simulink model "Roboter_RRP_Sim"  (R2020b)
settings: Solver=ode15s  StartTime=0.0  StopTime=5  RelTol=1e-6  AbsTol=1e-5  EnableMultiTasking=on
InitFcn:
  | set_parameter
StartFcn:
  | set_parameter
undefined symbols (not defined in the file or in its folder): parReg, parSys, X, Y, Z
libraries: sm_lib x14, nesl_utility x4, fl_lib x1
settings Model: Creator=andreas  LastModifiedBy=ukn
settings SolverCC: AutoScaleAbsTol=off  MaxOrder=3
settings DataIOCC: LimitDataPoints=on  SaveFormat=Array  SignalLoggingSaveFormat=ModelDataLogs  ReturnWorkspaceOutputs=off
settings OptimizationCC: ExpressionDepthLimit=2147483647  InitFltsAndDblsToZero=on  LifeSpan=inf
settings DebuggingCC: SaveWithParameterizedLinksMsg=none  UnderspecifiedInitializationDetection=Classic  MergeDetectMultiDrivingBlocksExec=none  SignalResolutionControl=TryResolveAllWithWarning  SolverPrmCheckMsg=warning  MultiTaskDSMMsg=warning  MultiTaskCondExecSysMsg=none  FcnCallInpInsideContextMsg=warning  StateNameClashWarn=warning  SFUnexpectedBacktrackingDiag=warning  SFNoUnconditionalDefaultTransitionDiag=warning  SFExecutionAtInitializationDiag=none  ArithmeticOperatorsInVariantConditions=warning
settings HardwareCC: ProdBitPerPointer=32  ProdBitPerSizeT=32  ProdBitPerPtrDiffT=32  ProdLargestAtomicFloat=None  ProdIntDivRoundTo=Undefined  ProdEndianess=Unspecified  ProdWordSize=32  ProdHWDeviceType=32-bit Generic
settings ModelReferenceCC: PropagateSignalLabelsOutOfModel=off
settings SFSimCC: SimUseLocalCustomCode=off  CustomCodeUndefinedFunction=UseInterfaceOnly
settings RTWCC: RTWUseLocalCustomCode=off
settings CodeAppCC: StateflowObjectComments=on
settings GRTTargetCC: TargetFcnLib=ansi_tfl_tmw.mat  TargetLangStandard=C89/C90 (ANSI)  CombineOutputUpdateFcns=off  GRTInterface=on
settings ConfigComp: CovMetricSettings=dw  CovSaveCumulativeToWorkspaceVar=on  CovSaveSingleToWorkspaceVar=on  CovExternalEMLEnable=off

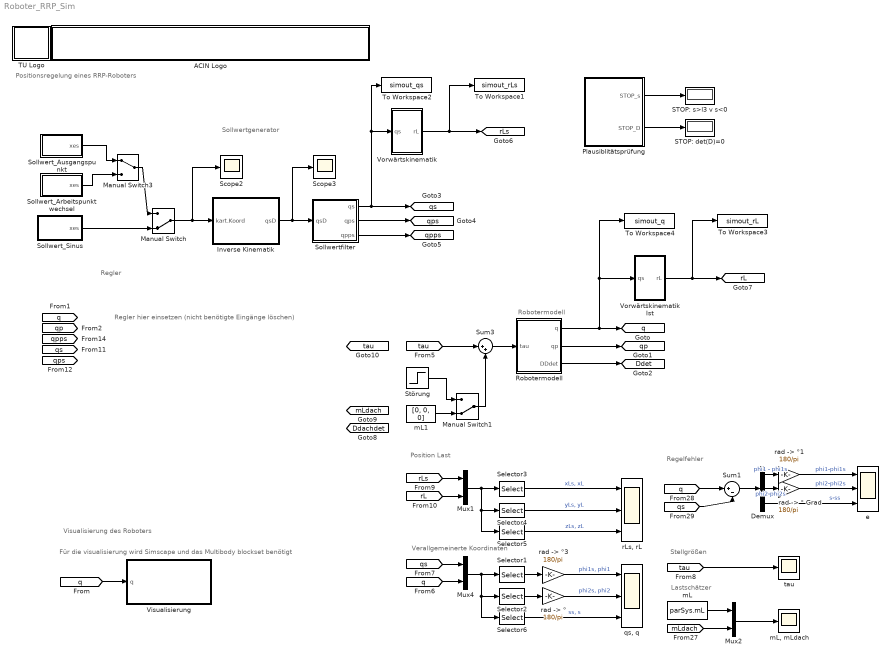
== system Roboter_RRP_Sim ==
  note: Positionsregelung eines RRP-Roboters
  note: Robotermodell
  note: Regler
  note: Sollwertgenerator
  note: Position Last
  note: Verallgemeinerte Koordinaten
  note: Regelfehler
  note: Stellgrößen
  note: Lastschätzer
  note: Regler
      | hier
      | einsetzen
      | (nicht benötigte Eingänge löschen)
  note: Für die visualisierung wird Simscape und das Multibody blockset benötigt
  note: Visualisierung des Roboters
  ACIN Logo : Subsystem
      mask init:
      | s = get_param(gcb,'UserData');
      mask Display:
      | image(s.logo,[0 0 439 45]);
      | %axis image
  Demux : Demux  Outputs=3
  Inverse Kinematik : Subsystem
  Manual Switch : ManualSwitch  CurrentSetting=0
  Manual Switch1 : ManualSwitch  CurrentSetting=0
  Manual Switch3 : ManualSwitch
  Mux1 : Mux  Inputs=2
  Mux2 : Mux  Inputs=2
  Mux4 : Mux  Inputs=2
  Plausiblitätsprüfung : Subsystem
  Robotermodell : Subsystem
  STOP: det(D)=0 : Display
  STOP: s>l3 v s<0 : Display
  Scope2 : Scope
  Scope3 : Scope
  Selector1 : Selector  InputPortWidth=6  IndexOptions=Index vector (dialog)  Indices=[1 4]  OutputSizes=1
  Selector2 : Selector  InputPortWidth=6  IndexOptions=Index vector (dialog)  Indices=[2 5]  OutputSizes=1
  Selector3 : Selector  InputPortWidth=6  IndexOptions=Index vector (dialog)  Indices=[1 4]  OutputSizes=1
  Selector4 : Selector  InputPortWidth=6  IndexOptions=Index vector (dialog)  Indices=[2 5]  OutputSizes=1
  Selector5 : Selector  InputPortWidth=6  IndexOptions=Index vector (dialog)  Indices=[3 6]  OutputSizes=1
  Selector6 : Selector  InputPortWidth=6  IndexOptions=Index vector (dialog)  Indices=[3 6]  OutputSizes=1
  Sollwert_Arbeitspunktwechsel : Subsystem
  Sollwert_Ausgangspunkt : Subsystem
  Sollwert_Sinus : Subsystem
  Sollwertfilter : Subsystem
  Störung : Step  After=[250, 250, 200]  SampleTime=0
  Sum1 : Sum  Inputs=|+-
  Sum3 : Sum  Inputs=|++
  TU Logo : Subsystem
      mask init:
      | s = get_param(gcb,'UserData');
      mask Display: image(s.logo,[0 0 45 45]);
  To Workspace1 : ToWorkspace  VariableName=simout_rLs  SaveFormat=Structure With Time  SampleTime=-1
  To Workspace2 : ToWorkspace  VariableName=simout_qs  SaveFormat=Structure With Time  SampleTime=-1
  To Workspace3 : ToWorkspace  VariableName=simout_rL  SaveFormat=Structure With Time  SampleTime=-1
  To Workspace4 : ToWorkspace  VariableName=simout_q  SaveFormat=Structure With Time  SampleTime=-1
  Visualisierung : Subsystem
  Vorwärtskinematik : Subsystem
  Vorwärtskinematik Ist : Subsystem
  e : Scope  NumInputPorts=3
  mL : Constant  Value=parSys.mL
  "mL, mLdach" : Scope
  mL1 : Constant  Value=[0, 0, 0]
  "qs, q" : Scope  NumInputPorts=3
  "rLs, rL" : Scope  NumInputPorts=3
  "rad -> °" : Gain  Gain=180/pi
  "rad -> ° Grad" : Gain  Gain=180/pi
  "rad -> °1" : Gain  Gain=180/pi
  "rad -> °3" : Gain  Gain=180/pi
  tau : Scope
  tag scope: Ddachdet=global, Ddet=global, mLdach=global, q=global, qp=global, qpps=global, qps=global, qs=global, rL=global, rLs=global, tau=global
  wires:
  Robotermodell/1(q) -> Vorwärtskinematik Ist/1(qs), To Workspace4/1, [q]
  Robotermodell/2(qp) -> [qp]
  Inverse Kinematik/1(qsD) -> Scope3/1, Sollwertfilter/1(qsD)
  [tau] -> tau/1
  Vorwärtskinematik Ist/1(rL) -> [rL], To Workspace3/1
  Manual Switch/1 -> Inverse Kinematik/1(kart.Koord), Scope2/1
  Sollwert_Sinus/1(xes) -> Manual Switch/2
  [qs] -> Mux4/1
  [q] -> Mux4/2
  Mux4/1 -> Selector1/1, Selector2/1, Selector6/1
  [rLs] -> Mux1/1
  [rL] -> Mux1/2
  Selector3/1 -> "rLs, rL"/1  "xLs, xL"
  Selector4/1 -> "rLs, rL"/2  "yLs, yL"
  Selector5/1 -> "rLs, rL"/3  "zLs, zL"
  Mux1/1 -> Selector5/1, Selector4/1, Selector3/1
  Manual Switch3/1 -> Manual Switch/1
  Sollwert_Arbeitspunktwechsel/1(xes) -> Manual Switch3/2
  Sollwert_Ausgangspunkt/1(xes) -> Manual Switch3/1
  Plausiblitätsprüfung/1(STOP_s) -> STOP: s>l3 v s<0/1
  Sollwertfilter/1(qs) -> [qs], Vorwärtskinematik/1(qs), To Workspace2/1
  Sollwertfilter/3(qpps) -> [qpps]
  Sollwertfilter/2(qps) -> [qps]
  [q] -> Sum1/1
  Demux/1 -> "rad -> °1"/1  "phi1 - phi1s"
  Demux/2 -> "rad -> ° Grad"/1  "phi2-phi2s"
  Demux/3 -> e/3  "s-ss"
  [qs] -> Sum1/2
  Sum1/1 -> Demux/1
  [tau] -> Sum3/1
  Sum3/1 -> Robotermodell/1(tau)
  Störung/1 -> Manual Switch1/1
  mL1/1 -> Manual Switch1/2
  Manual Switch1/1 -> Sum3/2
  Mux2/1 -> "mL, mLdach"/1
  mL/1 -> Mux2/1
  [mLdach] -> Mux2/2
  Selector1/1 -> "rad -> °3"/1
  Selector2/1 -> "rad -> °"/1
  Selector6/1 -> "qs, q"/3  "ss, s"
  "rad -> °"/1 -> "qs, q"/2  "phi2s, phi2"
  "rad -> °3"/1 -> "qs, q"/1  "phi1s, phi1"
  "rad -> °1"/1 -> e/1  "phi1-phi1s"
  "rad -> ° Grad"/1 -> e/2  "phi2-phi2s"
  Vorwärtskinematik/1(rL) -> [rLs], To Workspace1/1
  Plausiblitätsprüfung/2(STOP_D) -> STOP: det(D)=0/1
  Robotermodell/3(DDdet) -> [Ddet]
  [q] -> Visualisierung/1(q)

== system Roboter_RRP_Sim/ACIN Logo ==

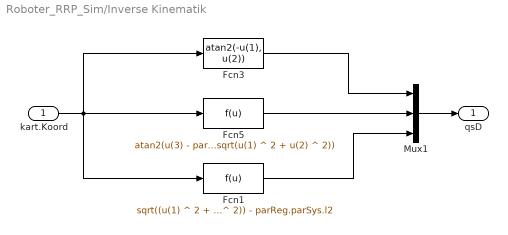
== system Roboter_RRP_Sim/Inverse Kinematik ==
  kart.Koord : Inport
  Fcn1 : Fcn  Expr=sqrt((u(1) ^ 2 + u(2) ^ 2 + u(3) ^ 2 - 2 * u(3) * parReg.parSys.l1 + parReg.parSys.l1 ^ 2)) - parReg.parSys.l2
  Fcn3 : Fcn  Expr=atan2(-u(1), u(2))
  Fcn5 : Fcn  Expr=atan2(u(3) - parReg.parSys.l1, sqrt(u(1) ^ 2 + u(2) ^ 2))
  Mux1 : Mux  Inputs=3
  qsD : Outport
  wires:
  kart.Koord/1 -> Fcn3/1, Fcn1/1, Fcn5/1
  Fcn3/1 -> Mux1/1
  Fcn5/1 -> Mux1/2
  Mux1/1 -> qsD/1
  Fcn1/1 -> Mux1/3

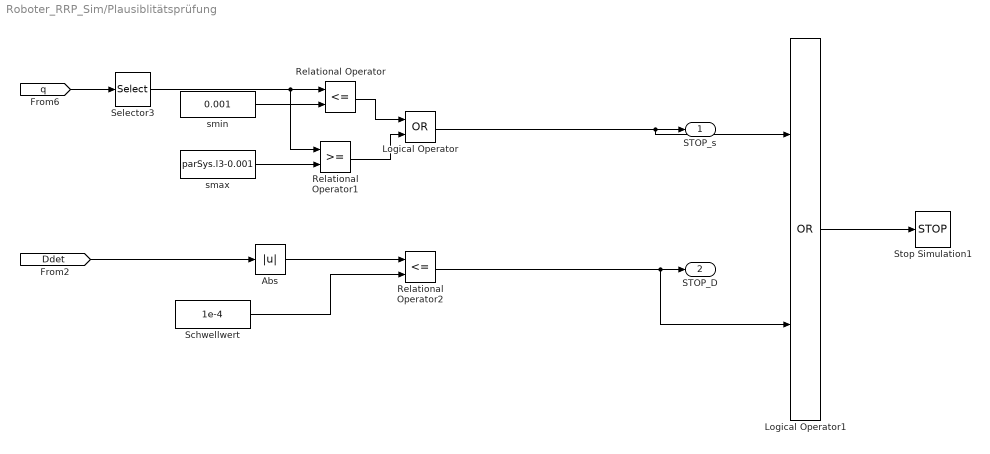
== system Roboter_RRP_Sim/Plausiblitätsprüfung ==
  Abs : Abs
  Logical Operator : Logic  Operator=OR  AllPortsSameDT=off  OutDataTypeStr=boolean
  Logical Operator1 : Logic  Operator=OR  AllPortsSameDT=off  OutDataTypeStr=boolean
  Relational Operator : RelationalOperator  Operator=<=  OutDataTypeStr=boolean  RndMeth=Nearest
  Relational Operator1 : RelationalOperator  OutDataTypeStr=boolean  RndMeth=Nearest
  Relational Operator2 : RelationalOperator  Operator=<=  OutDataTypeStr=boolean  RndMeth=Nearest
  Schwellwert : Constant  Value=1e-4
  Selector3 : Selector  InputPortWidth=3  IndexOptions=Index vector (dialog)  Indices=[3]  OutputSizes=1
  Stop Simulation1 : Stop
  smax : Constant  Value=parSys.l3-0.001
  smin : Constant  Value=0.001
  STOP_s : Outport
  STOP_D : Outport  Port=2
  wires:
  Relational Operator/1 -> Logical Operator/1
  Relational Operator1/1 -> Logical Operator/2
  [q] -> Selector3/1
  Selector3/1 -> Relational Operator/1, Relational Operator1/1
  smin/1 -> Relational Operator/2
  [Ddet] -> Abs/1
  Abs/1 -> Relational Operator2/1
  Schwellwert/1 -> Relational Operator2/2
  Logical Operator1/1 -> Stop Simulation1/1
  smax/1 -> Relational Operator1/2
  Relational Operator2/1 -> STOP_D/1, Logical Operator1/2
  Logical Operator/1 -> STOP_s/1, Logical Operator1/1

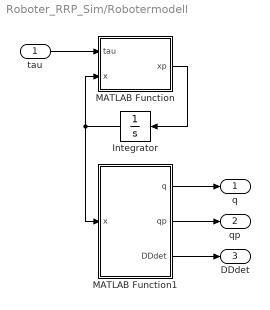
== system Roboter_RRP_Sim/Robotermodell ==
  tau : Inport
  Integrator : Integrator  InitialCondition=[parSys.phi10; parSys.phi20; parSys.s0; parSys.phi1p0; parSys.phi2p0; parSys.sp0]
  MATLAB Function : MATLAB Function  TreatAsAtomicUnit=on
  MATLAB Function1 : MATLAB Function  TreatAsAtomicUnit=on
  q : Outport
  qp : Outport  Port=2
  DDdet : Outport  Port=3
  wires:
  MATLAB Function1/2(qp) -> qp/1
  MATLAB Function/1(xp) -> Integrator/1
  MATLAB Function1/3(DDdet) -> DDdet/1
  Integrator/1 -> MATLAB Function1/1(x), MATLAB Function/2(x)
  tau/1 -> MATLAB Function/1(tau)
  MATLAB Function1/1(q) -> q/1

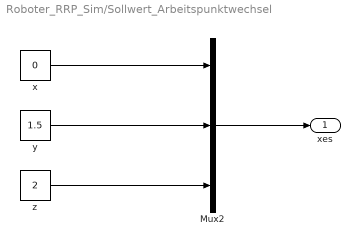
== system Roboter_RRP_Sim/Sollwert_Arbeitspunktwechsel ==
  Mux2 : Mux  Inputs=3
  x : Constant  Value=0
  y : Constant  Value=1.5
  z : Constant  Value=2
  xes : Outport
  wires:
  Mux2/1 -> xes/1
  x/1 -> Mux2/1
  y/1 -> Mux2/2
  z/1 -> Mux2/3

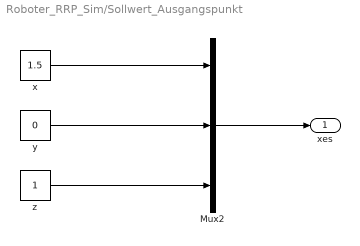
== system Roboter_RRP_Sim/Sollwert_Ausgangspunkt ==
  Mux2 : Mux  Inputs=3
  x : Constant  Value=1.5
  y : Constant  Value=0
  z : Constant
  xes : Outport
  wires:
  z/1 -> Mux2/3
  y/1 -> Mux2/2
  x/1 -> Mux2/1
  Mux2/1 -> xes/1

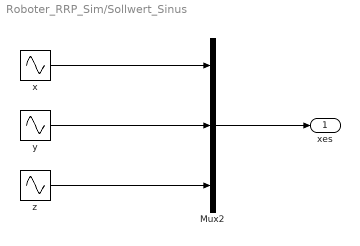
== system Roboter_RRP_Sim/Sollwert_Sinus ==
  Mux2 : Mux  Inputs=3
  x : Sin  Amplitude=1.5  Frequency=2*pi*parReg.traj_fKreis  Phase=pi/2  SampleTime=0
  y : Sin  Amplitude=1.5  Frequency=2*pi*parReg.traj_fKreis  SampleTime=0
  z : Sin  Amplitude=0.5  Bias=1.5  Frequency=2*pi*parReg.traj_fz  Phase=-pi/2  SampleTime=0
  xes : Outport
  wires:
  Mux2/1 -> xes/1
  x/1 -> Mux2/1
  y/1 -> Mux2/2
  z/1 -> Mux2/3

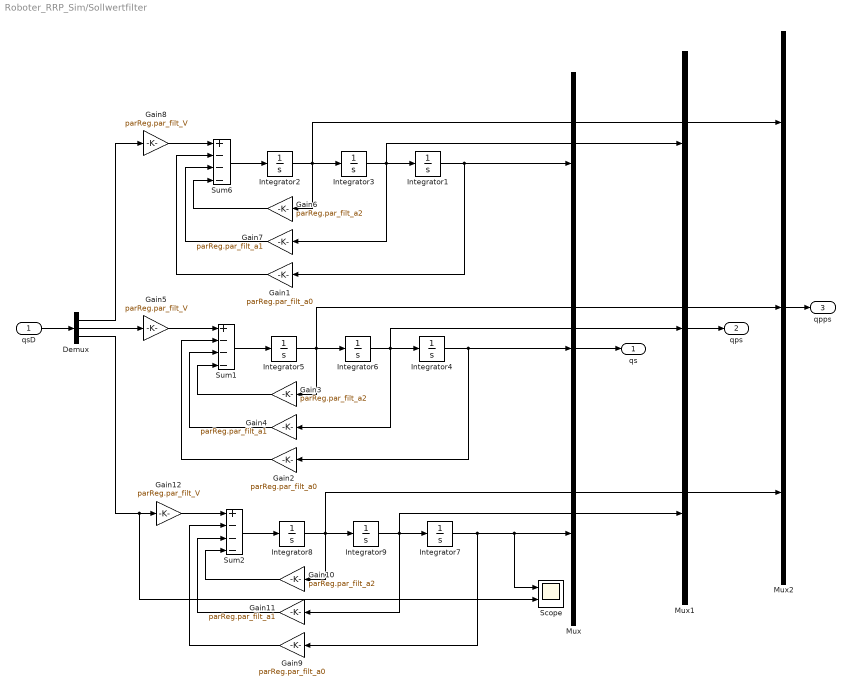
== system Roboter_RRP_Sim/Sollwertfilter ==
  qsD : Inport
  Demux : Demux  Outputs=3
  Gain1 : Gain  Gain=parReg.par_filt_a0  SaturateOnIntegerOverflow=on  OutDataTypeStr=Inherit: Same as input  ParamDataTypeStr=Inherit: Same as input
  Gain10 : Gain  Gain=parReg.par_filt_a2  SaturateOnIntegerOverflow=on  OutDataTypeStr=Inherit: Same as input  ParamDataTypeStr=Inherit: Same as input
  Gain11 : Gain  Gain=parReg.par_filt_a1  SaturateOnIntegerOverflow=on  OutDataTypeStr=Inherit: Same as input  ParamDataTypeStr=Inherit: Same as input
  Gain12 : Gain  Gain=parReg.par_filt_V  SaturateOnIntegerOverflow=on  OutDataTypeStr=Inherit: Same as input  ParamDataTypeStr=Inherit: Same as input
  Gain2 : Gain  Gain=parReg.par_filt_a0  SaturateOnIntegerOverflow=on  OutDataTypeStr=Inherit: Same as input  ParamDataTypeStr=Inherit: Same as input
  Gain3 : Gain  Gain=parReg.par_filt_a2  SaturateOnIntegerOverflow=on  OutDataTypeStr=Inherit: Same as input  ParamDataTypeStr=Inherit: Same as input
  Gain4 : Gain  Gain=parReg.par_filt_a1  SaturateOnIntegerOverflow=on  OutDataTypeStr=Inherit: Same as input  ParamDataTypeStr=Inherit: Same as input
  Gain5 : Gain  Gain=parReg.par_filt_V  SaturateOnIntegerOverflow=on  OutDataTypeStr=Inherit: Same as input  ParamDataTypeStr=Inherit: Same as input
  Gain6 : Gain  Gain=parReg.par_filt_a2  SaturateOnIntegerOverflow=on  OutDataTypeStr=Inherit: Same as input  ParamDataTypeStr=Inherit: Same as input
  Gain7 : Gain  Gain=parReg.par_filt_a1  SaturateOnIntegerOverflow=on  OutDataTypeStr=Inherit: Same as input  ParamDataTypeStr=Inherit: Same as input
  Gain8 : Gain  Gain=parReg.par_filt_V  SaturateOnIntegerOverflow=on  OutDataTypeStr=Inherit: Same as input  ParamDataTypeStr=Inherit: Same as input
  Gain9 : Gain  Gain=parReg.par_filt_a0  SaturateOnIntegerOverflow=on  OutDataTypeStr=Inherit: Same as input  ParamDataTypeStr=Inherit: Same as input
  Integrator1 : Integrator  InitialCondition=parReg.traj_phi10
  Integrator{2..3,5..6,8..9} (6 alike) : Integrator
  Integrator4 : Integrator  InitialCondition=parReg.traj_phi20
  Integrator7 : Integrator  InitialCondition=parReg.traj_s0
  Mux : Mux  Inputs=3
  Mux1 : Mux  Inputs=3
  Mux2 : Mux  Inputs=3
  Scope : Scope  NumInputPorts=2
  Sum1 : Sum  Inputs=+---  InputSameDT=on  SaturateOnIntegerOverflow=on  OutDataTypeStr=Inherit: Same as first input
  Sum2 : Sum  Inputs=+---  InputSameDT=on  SaturateOnIntegerOverflow=on  OutDataTypeStr=Inherit: Same as first input
  Sum6 : Sum  Inputs=+---  InputSameDT=on  SaturateOnIntegerOverflow=on  OutDataTypeStr=Inherit: Same as first input
  qs : Outport
  qps : Outport  Port=2
  qpps : Outport  Port=3
  wires:
  Mux/1 -> qs/1
  qsD/1 -> Demux/1
  Demux/1 -> Gain8/1
  Sum6/1 -> Integrator2/1
  Gain8/1 -> Sum6/1
  Integrator3/1 -> Integrator1/1, Gain7/1, Mux1/1
  Integrator2/1 -> Integrator3/1, Gain6/1, Mux2/1
  Integrator1/1 -> Gain1/1, Mux/1
  Gain6/1 -> Sum6/4
  Gain7/1 -> Sum6/3
  Gain1/1 -> Sum6/2
  Sum1/1 -> Integrator5/1
  Gain5/1 -> Sum1/1
  Integrator6/1 -> Gain4/1, Integrator4/1, Mux1/2
  Integrator5/1 -> Gain3/1, Integrator6/1, Mux2/2
  Integrator4/1 -> Gain2/1, Mux/2
  Gain3/1 -> Sum1/4
  Gain4/1 -> Sum1/3
  Gain2/1 -> Sum1/2
  Demux/2 -> Gain5/1
  Sum2/1 -> Integrator8/1
  Gain12/1 -> Sum2/1
  Integrator9/1 -> Integrator7/1, Gain11/1, Mux1/3
  Integrator8/1 -> Integrator9/1, Gain10/1, Mux2/3
  Integrator7/1 -> Gain9/1, Mux/3, Scope/1
  Gain10/1 -> Sum2/4
  Gain11/1 -> Sum2/3
  Gain9/1 -> Sum2/2
  Demux/3 -> Gain12/1, Scope/2
  Mux1/1 -> qps/1
  Mux2/1 -> qpps/1

== system Roboter_RRP_Sim/TU Logo ==

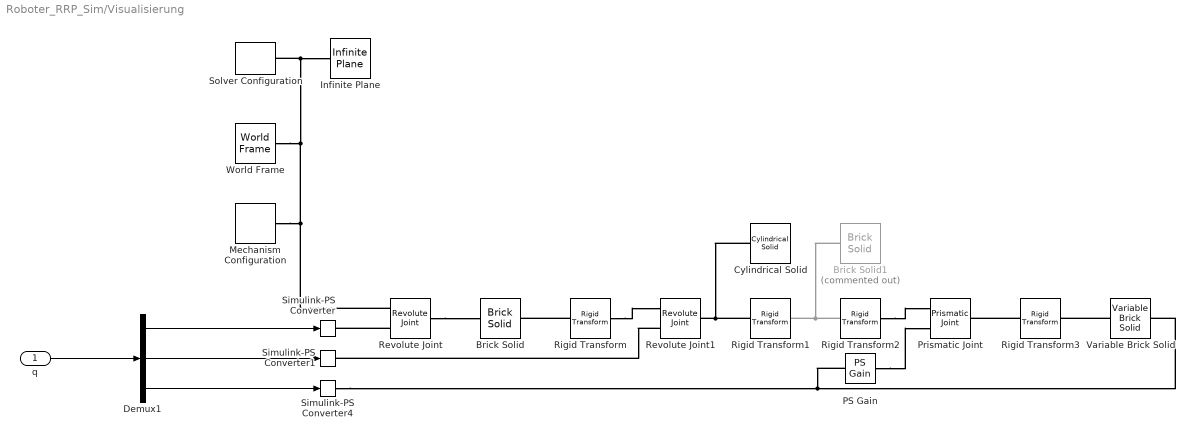
== system Roboter_RRP_Sim/Visualisierung ==
  q : Inport
  Brick Solid : sm_lib/Body Elements/Brick Solid  GraphicAmbientColor=[0.15 0.15 0.15 1.0]  BasedOnType=Density  BrickDimensions=[.1 .05 1]  BrickDimensionUnits=m  CenterOfMass=[0 0 0]  CenterOfMassUnits=m  GraphicDiffuseColor=[0.5 0.5 0.5]  Density=1000  DensityUnits=kg/m^3  DoExposeReferenceFrame=off  GraphicEmissiveColor=[0.0 0.0 0.0 1.0]  ExportEntireGeometry=off  SerializedFrames=<Frames><Frame><Id>Frame1</Id><Value><Name>F1</Name><Origin><Source>GeometricFeature</Source><FeatureName>-z surface</FeatureName></Origin><PrimaryAxis><DefinedDirection>+Z</DefinedDirection><Source>ReferenceFrame</Source><SourceDirection>+Z</SourceDirection><FeatureName></FeatureName></PrimaryAxis><SecondaryAxis><DefinedDirection>+X</DefinedDirection><Source>ReferenceFrame</Source><SourceDirection>+X</SourceDirection><FeatureName></FeatureName></SecondaryAxis></Value></Frame><Frame><Id>Frame2</Id><Value><Name>F2</Name><Origin><Source>GeometricFeature</Source><FeatureName>+z surface</FeatureName></Origin><PrimaryAxis><DefinedDirection>+Z</DefinedDirection><Source>ReferenceFrame</Source><SourceDirection>+Z</SourceDirection><FeatureName></FeatureName></PrimaryAxis><SecondaryAxis><DefinedDirection>+X</DefinedDirection><Source>ReferenceFrame</Source><SourceDirection>+X</SourceDirection><FeatureName></FeatureName></SecondaryAxis></Value></Frame></Frames>  MarkerShape=Sphere  MarkerSize=10  GraphicType=FromGeometry  InertiaType=CalculateFromGeometry  Mass=1  MassUnits=kg  MomentsOfInertia=[1 1 1]  MomentsOfInertiaUnits=kg*m^2  GraphicOpacity=1.0  ProductsOfInertia=[0 0 0]  ProductsOfInertiaUnits=kg*m^2  GraphicShininess=75  GraphicSpecularColor=[0.5 0.5 0.5 1.0]  GraphicVisPropType=SimpleVisualProperties
  Brick Solid1 : sm_lib/Body Elements/Brick Solid  Commented=on  GraphicAmbientColor=[0.15 0.15 0.15 1.0]  BasedOnType=Density  BrickDimensions=[.1 .5 .05]  BrickDimensionUnits=m  CenterOfMass=[0 0 0]  CenterOfMassUnits=m  GraphicDiffuseColor=[0.5 0.5 0.5]  Density=1000  DensityUnits=kg/m^3  DoExposeReferenceFrame=off  GraphicEmissiveColor=[0.0 0.0 0.0 1.0]  ExportEntireGeometry=off  SerializedFrames=<Frames><Frame><Id>Frame1</Id><Value><Name>F1</Name><Origin><Source>GeometricFeature</Source><FeatureName>-y surface</FeatureName></Origin><PrimaryAxis><DefinedDirection>+Z</DefinedDirection><Source>ReferenceFrame</Source><SourceDirection>+Z</SourceDirection><FeatureName></FeatureName></PrimaryAxis><SecondaryAxis><DefinedDirection>+X</DefinedDirection><Source>ReferenceFrame</Source><SourceDirection>+X</SourceDirection><FeatureName></FeatureName></SecondaryAxis></Value></Frame><Frame><Id>Frame2</Id><Value><Name>F2</Name><Origin><Source>GeometricFeature</Source><FeatureName>+y surface</FeatureName></Origin><PrimaryAxis><DefinedDirection>+Z</DefinedDirection><Source>ReferenceFrame</Source><SourceDirection>+Z</SourceDirection><FeatureName></FeatureName></PrimaryAxis><SecondaryAxis><DefinedDirection>+X</DefinedDirection><Source>ReferenceFrame</Source><SourceDirection>+X</SourceDirection><FeatureName></FeatureName></SecondaryAxis></Value></Frame></Frames>  MarkerShape=Sphere  MarkerSize=10  GraphicType=FromGeometry  InertiaType=CalculateFromGeometry  Mass=1  MassUnits=kg  MomentsOfInertia=[1 1 1]  MomentsOfInertiaUnits=kg*m^2  GraphicOpacity=1.0  ProductsOfInertia=[0 0 0]  ProductsOfInertiaUnits=kg*m^2  GraphicShininess=75  GraphicSpecularColor=[0.5 0.5 0.5 1.0]  GraphicVisPropType=SimpleVisualProperties
  Cylindrical Solid : sm_lib/Body Elements/Cylindrical Solid  GraphicAmbientColor=[0.15 0.15 0.15 1.0]  BasedOnType=Density  CenterOfMass=[0 0 0]  CenterOfMassUnits=m  GraphicDiffuseColor=[0.5 0.5 0.5]  CylinderLength=.1  CylinderLengthUnits=m  CylinderRadius=.05  CylinderRadiusUnits=m  Density=1000  DensityUnits=kg/m^3  DoExposeReferenceFrame=on  GraphicEmissiveColor=[0.0 0.0 0.0 1.0]  ExportEntireGeometry=off  SerializedFrames=<Frames/>  MarkerShape=Sphere  MarkerSize=10  GraphicType=FromGeometry  InertiaType=CalculateFromGeometry  Mass=1  MassUnits=kg  MomentsOfInertia=[1 1 1]  MomentsOfInertiaUnits=kg*m^2  GraphicOpacity=1.0  ProductsOfInertia=[0 0 0]  ProductsOfInertiaUnits=kg*m^2  GraphicShininess=75  GraphicSpecularColor=[0.5 0.5 0.5 1.0]  GraphicVisPropType=SimpleVisualProperties
  Demux1 : Demux  Outputs=3
  Infinite Plane : sm_lib/Curves and Surfaces/Infinite Plane  GraphicType=Rectangle  GraphicPlaneWidth=1  GraphicPlaneWidthUnits=m  GraphicPlaneHeight=1  GraphicPlaneHeightUnits=m  GraphicVisPropType=SimpleVisualProperties  GraphicDiffuseColor=[0.5 0.5 0.5]  GraphicOpacity=0.25  GraphicSpecularColor=[0.5 0.5 0.5 1.0]  GraphicAmbientColor=[0.15 0.15 0.15 1.0]  GraphicEmissiveColor=[0.0 0.0 0.0 1.0]  GraphicShininess=75
  Mechanism Configuration : sm_lib/Utilities/Mechanism Configuration  UniformGravity=Constant  GravityVector=[0 0 0]  GravityVectorUnits=m/s^2  GravityUnits=m/s^2  LinearizationDelta=0.001  JointModeTransitionNonlinearIterations=2
  PS Gain : fl_lib/Physical Signals/Functions/PS Gain  gain=.5
  Prismatic Joint : sm_lib/Joints/Prismatic Joint  JointMode=Normal  SenseConstraintForce=off  SenseConstraintForceX=off  SenseConstraintForceY=off  SenseConstraintForceZ=off  SenseConstraintTorque=off  SenseConstraintTorqueX=off  SenseConstraintTorqueY=off  SenseConstraintTorqueZ=off  SenseTotalForce=off  SenseTotalForceX=off  SenseTotalForceY=off  SenseTotalForceZ=off  SenseTotalTorque=off  SenseTotalTorqueX=off  SenseTotalTorqueY=off  SenseTotalTorqueZ=off  CompositeWrenchDir=FollowerOnBase  CompositeWrenchFrame=BaseFrame  EquilibriumPosition=0  EquilibriumPositionUnits=m  SpringStiffness=0  SpringStiffnessUnits=N/m  DampingCoefficient=0  DampingCoefficientUnits=N/(m/s)  TorqueActuationMode=ComputedTorque  MotionActuationMode=InputMotion  SensePosition=off  SenseVelocity=off  SenseAcceleration=off  SenseTorqueForce=off  SenseLowerLimitTorqueForce=off  SenseUpperLimitTorqueForce=off  LowerLimitSpecify=off  LowerLimitBound=-1  LowerLimitBoundUnits=m  LowerLimitStiffness=1e6  LowerLimitStiffnessUnits=N/m  LowerLimitDamping=1e3  LowerLimitDampingUnits=N/(m/s)  LowerLimitTransitionRegionWidth=1e-4  LowerLimitTransitionRegionWidthUnits=m  UpperLimitSpecify=off  UpperLimitBound=1  UpperLimitBoundUnits=m  UpperLimitStiffness=1e6  UpperLimitStiffnessUnits=N/m  UpperLimitDamping=1e3  UpperLimitDampingUnits=N/(m/s)  UpperLimitTransitionRegionWidth=1e-4  UpperLimitTransitionRegionWidthUnits=m  PositionTargetSpecify=off  PositionTargetPriority=High  PositionTargetValue=0  PositionTargetValueUnits=m  VelocityTargetSpecify=off  VelocityTargetPriority=High  VelocityTargetValue=0  VelocityTargetValueUnits=m/s
  Revolute Joint : sm_lib/Joints/Revolute Joint  JointMode=Normal  SenseConstraintForce=off  SenseConstraintForceX=off  SenseConstraintForceY=off  SenseConstraintForceZ=off  SenseConstraintTorque=off  SenseConstraintTorqueX=off  SenseConstraintTorqueY=off  SenseConstraintTorqueZ=off  SenseTotalForce=off  SenseTotalForceX=off  SenseTotalForceY=off  SenseTotalForceZ=off  SenseTotalTorque=off  SenseTotalTorqueX=off  SenseTotalTorqueY=off  SenseTotalTorqueZ=off  CompositeWrenchDir=FollowerOnBase  CompositeWrenchFrame=BaseFrame  EquilibriumPosition=0  EquilibriumPositionUnits=deg  SpringStiffness=0  SpringStiffnessUnits=N*m/deg  DampingCoefficient=0  DampingCoefficientUnits=N*m/(deg/s)  TorqueActuationMode=ComputedTorque  MotionActuationMode=InputMotion  SensePosition=off  SenseVelocity=off  SenseAcceleration=off  SenseTorqueForce=off  SenseLowerLimitTorqueForce=off  SenseUpperLimitTorqueForce=off  LowerLimitSpecify=off  LowerLimitBound=-90  LowerLimitBoundUnits=deg  LowerLimitStiffness=1e4  LowerLimitStiffnessUnits=N*m/deg  LowerLimitDamping=10  LowerLimitDampingUnits=N*m/(deg/s)  LowerLimitTransitionRegionWidth=0.1  LowerLimitTransitionRegionWidthUnits=deg  UpperLimitSpecify=off  UpperLimitBound=90  UpperLimitBoundUnits=deg  UpperLimitStiffness=1e4  UpperLimitStiffnessUnits=N*m/deg  UpperLimitDamping=10  UpperLimitDampingUnits=N*m/(deg/s)  UpperLimitTransitionRegionWidth=0.1  UpperLimitTransitionRegionWidthUnits=deg  PositionTargetSpecify=off  PositionTargetPriority=High  PositionTargetValue=0  PositionTargetValueUnits=deg  VelocityTargetSpecify=off  VelocityTargetPriority=High  VelocityTargetValue=0  VelocityTargetValueUnits=deg/s
  Revolute Joint1 : sm_lib/Joints/Revolute Joint  JointMode=Normal  SenseConstraintForce=off  SenseConstraintForceX=off  SenseConstraintForceY=off  SenseConstraintForceZ=off  SenseConstraintTorque=off  SenseConstraintTorqueX=off  SenseConstraintTorqueY=off  SenseConstraintTorqueZ=off  SenseTotalForce=off  SenseTotalForceX=off  SenseTotalForceY=off  SenseTotalForceZ=off  SenseTotalTorque=off  SenseTotalTorqueX=off  SenseTotalTorqueY=off  SenseTotalTorqueZ=off  CompositeWrenchDir=FollowerOnBase  CompositeWrenchFrame=BaseFrame  EquilibriumPosition=0  EquilibriumPositionUnits=deg  SpringStiffness=0  SpringStiffnessUnits=N*m/deg  DampingCoefficient=0  DampingCoefficientUnits=N*m/(deg/s)  TorqueActuationMode=ComputedTorque  MotionActuationMode=InputMotion  SensePosition=off  SenseVelocity=off  SenseAcceleration=off  SenseTorqueForce=off  SenseLowerLimitTorqueForce=off  SenseUpperLimitTorqueForce=off  LowerLimitSpecify=off  LowerLimitBound=-90  LowerLimitBoundUnits=deg  LowerLimitStiffness=1e4  LowerLimitStiffnessUnits=N*m/deg  LowerLimitDamping=10  LowerLimitDampingUnits=N*m/(deg/s)  LowerLimitTransitionRegionWidth=0.1  LowerLimitTransitionRegionWidthUnits=deg  UpperLimitSpecify=off  UpperLimitBound=90  UpperLimitBoundUnits=deg  UpperLimitStiffness=1e4  UpperLimitStiffnessUnits=N*m/deg  UpperLimitDamping=10  UpperLimitDampingUnits=N*m/(deg/s)  UpperLimitTransitionRegionWidth=0.1  UpperLimitTransitionRegionWidthUnits=deg  PositionTargetSpecify=off  PositionTargetPriority=High  PositionTargetValue=0  PositionTargetValueUnits=deg  VelocityTargetSpecify=off  VelocityTargetPriority=High  VelocityTargetValue=0  VelocityTargetValueUnits=deg/s
  Rigid Transform : sm_lib/Frames and Transforms/Rigid Transform  TranslationMethod=None  TranslationStandardOffset=0  TranslationLengthUnit=m  TranslationStandardAxis=+Z  TranslationCartesianOffset=[0 0 0]  TranslationROffset=0  TranslationROffsetUnits=m  TranslationZOffset=0  TranslationZOffsetUnits=m  TranslationThetaOffset=0  TranslationThetaOffsetUnits=deg  RotationMethod=StandardAxis  RotationAngleUnits=deg  RotationStandardAxis=+Y  RotationAngle=90  RotationArbitraryAxis=[0 0 1]  FollAlignAxisA=+Y  BaseAlignAxisA=-X  FollAlignAxisB=+X  BaseAlignAxisB=+Z  RotationSequenceAxes=FollowerAxes  RotationSequence=XYX  RotationSequenceAngles=[0 0 0]  RotationSequenceAnglesUnits=deg  RotationMatrix=[1 0 0; 0 1 0; 0 0 1]
  Rigid Transform1 : sm_lib/Frames and Transforms/Rigid Transform  TranslationMethod=None  TranslationStandardOffset=0  TranslationLengthUnit=m  TranslationStandardAxis=+Z  TranslationCartesianOffset=[0 0 0]  TranslationROffset=0  TranslationROffsetUnits=m  TranslationZOffset=0  TranslationZOffsetUnits=m  TranslationThetaOffset=0  TranslationThetaOffsetUnits=deg  RotationMethod=StandardAxis  RotationAngleUnits=deg  RotationStandardAxis=+Y  RotationAngle=-90  RotationArbitraryAxis=[0 0 1]  FollAlignAxisA=+X  BaseAlignAxisA=+Y  FollAlignAxisB=+Y  BaseAlignAxisB=+Z  RotationSequenceAxes=FollowerAxes  RotationSequence=XYX  RotationSequenceAngles=[0 0 0]  RotationSequenceAnglesUnits=deg  RotationMatrix=[1 0 0; 0 1 0; 0 0 1]
  Rigid Transform2 : sm_lib/Frames and Transforms/Rigid Transform  TranslationMethod=None  TranslationStandardOffset=0  TranslationLengthUnit=m  TranslationStandardAxis=+Z  TranslationCartesianOffset=[0 0 0]  TranslationROffset=0  TranslationROffsetUnits=m  TranslationZOffset=0  TranslationZOffsetUnits=m  TranslationThetaOffset=0  TranslationThetaOffsetUnits=deg  RotationMethod=StandardAxis  RotationAngleUnits=deg  RotationStandardAxis=+X  RotationAngle=-90  RotationArbitraryAxis=[0 0 1]  FollAlignAxisA=+X  BaseAlignAxisA=+Y  FollAlignAxisB=+Y  BaseAlignAxisB=+Z  RotationSequenceAxes=FollowerAxes  RotationSequence=XYX  RotationSequenceAngles=[0 0 0]  RotationSequenceAnglesUnits=deg  RotationMatrix=[1 0 0; 0 1 0; 0 0 1]
  Rigid Transform3 : sm_lib/Frames and Transforms/Rigid Transform  TranslationMethod=StandardAxis  TranslationStandardOffset=.025  TranslationLengthUnit=m  TranslationStandardAxis=+Y  TranslationCartesianOffset=[0 0 0]  TranslationROffset=0  TranslationROffsetUnits=m  TranslationZOffset=0  TranslationZOffsetUnits=m  TranslationThetaOffset=0  TranslationThetaOffsetUnits=deg  RotationMethod=StandardAxis  RotationAngleUnits=deg  RotationStandardAxis=-X  RotationAngle=-90  RotationArbitraryAxis=[0 0 1]  FollAlignAxisA=+X  BaseAlignAxisA=+Y  FollAlignAxisB=+Y  BaseAlignAxisB=+Z  RotationSequenceAxes=FollowerAxes  RotationSequence=XYX  RotationSequenceAngles=[0 0 0]  RotationSequenceAnglesUnits=deg  RotationMatrix=[1 0 0; 0 1 0; 0 0 1]
  Simulink-PS Converter : nesl_utility/Simulink-PS Converter  PhysicalDomain=network_engine_domain  SubClassName=ps_input  LeftPortType=input  RightPortType=output  PseudoPeriodic=off  Frequencies=[]  NoiseDistribution=none  NoiseParameters=[]  Unit=1  AffineConversion=off  FilteringAndDerivatives=filter  SimscapeFilterOrder=2  InputFilterTimeConstant=0.001  UdotUserProvided=0
  Simulink-PS Converter1 : nesl_utility/Simulink-PS Converter  PhysicalDomain=network_engine_domain  SubClassName=ps_input  LeftPortType=input  RightPortType=output  PseudoPeriodic=off  Frequencies=[]  NoiseDistribution=none  NoiseParameters=[]  Unit=1  AffineConversion=off  FilteringAndDerivatives=filter  SimscapeFilterOrder=2  InputFilterTimeConstant=0.001  UdotUserProvided=0
  Simulink-PS Converter4 : nesl_utility/Simulink-PS Converter  PhysicalDomain=network_engine_domain  SubClassName=ps_input  LeftPortType=input  RightPortType=output  PseudoPeriodic=off  Frequencies=[]  NoiseDistribution=none  NoiseParameters=[]  Unit=1  AffineConversion=off  FilteringAndDerivatives=filter  SimscapeFilterOrder=2  InputFilterTimeConstant=0.001  UdotUserProvided=0
  Solver Configuration : nesl_utility/Solver Configuration  PhysicalDomain=network_engine_domain  SubClassName=solver  LeftPortType=input  RightPortType=generic  Tones=[]  Harmonics=[]  SimulateNoise=off  Profile=off  UseLocalSampling=off  EnableSwitchedLinearOptims=on  FrequencyDomain=off  UseCCode=off  RelTol=0.001  AbsTol=1e-06  MinStep=1e-09  ToWorkspace=off  RevertToSquareIcSolve=off  NumHomotopyIterations=100  PhasorMode=off  PhasorModeNumHarmonics=1  DoDC=off  ResidualTolerance=1e-09  UseLocalSolver=off  LocalSolverChoice=NE_BACKWARD_EULER_ADVANCER  LocalSolverSampleTime=0.001  DoFixedCost=off  MaxNonlinIter=3  MaxModeIter=2  ComputeImpulses=off  ImpulseIterations=2  LinearAlgebra=Sparse  EquationFormulation=NE_TIME_EF  DelaysMemoryBudget=1024  AutomaticFiltering=on  FilteringTimeConstant=0.001  PartitionStorageMethod=AS_NEEDED  PartitionMemoryBudget=1024  PartitionMethod=FAST
  Variable Brick Solid : sm_lib/Body Elements/Variable Mass/Variable Brick Solid  XLengthType=Constant  XLength=.1  XLengthUnits=m  YLengthType=ProvidedByInput  YLength=1  YLengthUnits=m  ZLengthType=Constant  ZLength=.05  ZLengthUnits=m  MassType=CalculateFromGeometry  InitialMassType=Specified  InitialMass=1  InitialMassUnits=kg  Density=1000  DensityUnits=kg/m^3  SenseXLength=off  SenseYLength=off  SenseZLength=off  SenseMass=off  SenseCenterOfMass=off  SenseInertiaMatrix=off  GraphicType=FromGeometry  MarkerShape=Sphere  MarkerSize=10  GraphicVisPropType=SimpleVisualProperties  GraphicDiffuseColor=[0.5 0.5 0.5]  GraphicSpecularColor=[0.5 0.5 0.5 1.0]  GraphicAmbientColor=[0.15 0.15 0.15 1.0]  GraphicEmissiveColor=[0.0 0.0 0.0 1.0]  GraphicShininess=75  GraphicOpacity=1.0
      settings: SourceProductBaseCode=MS
  World Frame : sm_lib/Frames and Transforms/World Frame
  wires:
  q/1 -> Demux1/1
  Demux1/2 -> Simulink-PS Converter1/1
  Demux1/1 -> Simulink-PS Converter/1
  Demux1/3 -> Simulink-PS Converter4/1
  connections:
  Revolute Joint/LConn2 -- Simulink-PS Converter/RConn1
  PS Gain/LConn1 -- Simulink-PS Converter4/RConn1 -- Variable Brick Solid/LConn1
  Revolute Joint/RConn1 -- Brick Solid/LConn1
  Rigid Transform/RConn1 -- Revolute Joint1/LConn1
  Variable Brick Solid/RConn1 -- Rigid Transform3/RConn1
  Revolute Joint1/LConn2 -- Simulink-PS Converter1/RConn1
  Rigid Transform/LConn1 -- Brick Solid/RConn1
  PS Gain/RConn1 -- Prismatic Joint/LConn2
  Solver Configuration/RConn1 -- Mechanism Configuration/RConn1 -- Revolute Joint/LConn1 -- World Frame/RConn1 -- Infinite Plane/LConn1
  Revolute Joint1/RConn1 -- Rigid Transform1/LConn1 -- Cylindrical Solid/RConn1
  Brick Solid1/LConn1 -- Rigid Transform1/RConn1 -- Rigid Transform2/LConn1
  Rigid Transform2/RConn1 -- Prismatic Joint/LConn1
  Rigid Transform3/LConn1 -- Prismatic Joint/RConn1

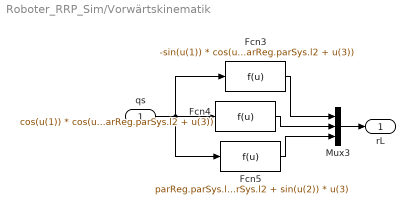
== system Roboter_RRP_Sim/Vorwärtskinematik ==
  qs : Inport
  Fcn3 : Fcn  Expr=-sin(u(1)) * cos(u(2)) * (parReg.parSys.l2 + u(3))
  Fcn4 : Fcn  Expr=cos(u(1)) * cos(u(2)) * (parReg.parSys.l2 + u(3))
  Fcn5 : Fcn  Expr=parReg.parSys.l1 + sin(u(2)) * parReg.parSys.l2 + sin(u(2)) * u(3)
  Mux3 : Mux  Inputs=3
  rL : Outport
  wires:
  Fcn3/1 -> Mux3/1
  Fcn4/1 -> Mux3/2
  Fcn5/1 -> Mux3/3
  qs/1 -> Fcn5/1, Fcn4/1, Fcn3/1
  Mux3/1 -> rL/1

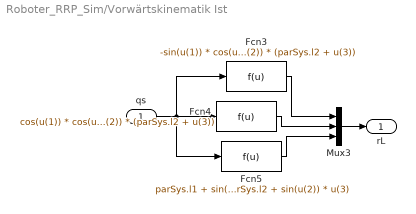
== system Roboter_RRP_Sim/Vorwärtskinematik Ist ==
  qs : Inport
  Fcn3 : Fcn  Expr=-sin(u(1)) * cos(u(2)) * (parSys.l2 + u(3))
  Fcn4 : Fcn  Expr=cos(u(1)) * cos(u(2)) * (parSys.l2 + u(3))
  Fcn5 : Fcn  Expr=parSys.l1 + sin(u(2)) * parSys.l2 + sin(u(2)) * u(3)
  Mux3 : Mux  Inputs=3
  rL : Outport
  wires:
  Mux3/1 -> rL/1
  qs/1 -> Fcn3/1, Fcn4/1, Fcn5/1
  Fcn5/1 -> Mux3/3
  Fcn4/1 -> Mux3/2
  Fcn3/1 -> Mux3/1

== matlab function Roboter_RRP_Sim/Robotermodell/MATLAB Function ==
  data: tau input; xp output; x input; parSys parameter
function xp = f(tau, x, parSys)

% define size of the output
xp = zeros(6,1);

% map parameters
m1  = parSys.m1;
m2  = parSys.m2;
m3  = parSys.m3;
mL  = parSys.mL;
l1  = parSys.l1;  
l2  = parSys.l2;  
l3  = parSys.l3;  
Ixx1 = parSys.Ixx1;  
Iyy1 = parSys.Iyy1;    
Izz1 = parSys.Izz1;  
Ixx2 = parSys.Ixx2;    
Iyy2 = parSys.Iyy2;    
Izz2 = parSys.Izz2;    
Ixx3 = parSys.Ixx3;    
Iyy3 = parSys.Iyy3;    
Izz3 = parSys.Izz3;    
d1   = parSys.d1;    
d2   = parSys.d2;    
d3   = parSys.d3; 
g    = parSys.g;

%  map inputs and states
M1   = tau(1);
M2   = tau(2);
F   =  tau(3);

phi1  = x(1);
phi2  = x(2);
s     = x(3);
phi1p = x(4);
phi2p = x(5);
sp    = x(6);


% inverse of the mass matrix
t1 = cos(phi2);
t1 = t1 ^ 2;
t2 = -0.4e1 + 0.4e1 * t1;
t3 = -8 * mL - 8 * m3;
t4 = l2 ^ 2;
t1 = Iyy2 * t2 + Iyy3 * t2 - t1 * (4 * mL * s ^ 2 + 4 * Izz2 + 4 * Izz3) - (4 * Izz1) - (m2 + 4 * m3 + 4 * mL) * t1 * t4 + t1 * (4 * l3 * m3 + s * t3) * l2 + t1 * (-l3 ^ 2 + (-4 * s + 4 * l3) * s) * m3;
t1 = 0.1e1 / t1;
t2 = m2 * t4 + m3 * ((l3 - 0.4e1 * l2) * l3 + ((4 * s) + 0.8e1 * l2 - (4 * l3)) * s + 0.4e1 * t4) + mL * (((4 * s) + 0.8e1 * l2) * s + 0.4e1 * t4) + (4 * Ixx2) + (4 * Ixx3);
t2 = 0.1e1 / t2;
t3 = -(t3 / 0.8e1);
t3 = 1 / t3;
DDinv = [-0.4e1 * t1 0 0; 0 0.4e1 * t2 0; 0 0 t3;];

% coriolis matrix C
CC = [cos(phi2) * (-phi2p * sin(phi2) * m2 * l2 ^ 2 - 0.4e1 * phi2p * sin(phi2) * m3 * l2 ^ 2 - 0.4e1 * phi2p * sin(phi2) * mL * l2 ^ 2 + 0.4e1 * phi2p * sin(phi2) * m3 * l2 * l3 - 0.8e1 * phi2p * sin(phi2) * m3 * l2 * s - 0.8e1 * phi2p * sin(phi2) * l2 * mL * s - phi2p * sin(phi2) * m3 * l3 ^ 2 + 0.4e1 * phi2p * sin(phi2) * m3 * s * l3 - 0.4e1 * phi2p * sin(phi2) * m3 * s ^ 2 - 0.4e1 * phi2p * sin(phi2) * Izz3 + 0.4e1 * phi2p * sin(phi2) * Iyy3 - 0.4e1 * phi2p * sin(phi2) * Izz2 + 0.4e1 * phi2p * sin(phi2) * Iyy2 - 0.4e1 * phi2p * sin(phi2) * mL * s ^ 2 + 0.4e1 * sp * cos(phi2) * m3 * s - 0.2e1 * sp * cos(phi2) * m3 * l3 + 0.4e1 * sp * cos(phi2) * m3 * l2 + 0.4e1 * sp * cos(phi2) * mL * l2 + 0.4e1 * sp * cos(phi2) * mL * s) / 0.4e1 (-m2 * l2 ^ 2 - 0.4e1 * m3 * l2 ^ 2 - 0.4e1 * mL * l2 ^ 2 + 0.4e1 * m3 * l2 * l3 - 0.8e1 * m3 * l2 * s - 0.8e1 * l2 * mL * s - m3 * l3 ^ 2 + 0.4e1 * m3 * s * l3 - 0.4e1 * m3 * s ^ 2 - 0.4e1 * Izz3 + 0.4e1 * Iyy3 - 0.4e1 * Izz2 + 0.4e1 * Iyy2 - 0.4e1 * mL * s ^ 2) * phi1p * sin(phi2) * cos(phi2) / 0.4e1 cos(phi2) ^ 2 * phi1p * (0.2e1 * m3 * s - m3 * l3 + 0.2e1 * m3 * l2 + 0.2e1 * mL * l2 + 0.2e1 * mL * s) / 0.2e1; -(-m2 * l2 ^ 2 - 0.4e1 * m3 * l2 ^ 2 - 0.4e1 * mL * l2 ^ 2 + 0.4e1 * m3 * l2 * l3 - 0.8e1 * m3 * l2 * s - 0.8e1 * l2 * mL * s - m3 * l3 ^ 2 + 0.4e1 * m3 * s * l3 - 0.4e1 * m3 * s ^ 2 - 0.4e1 * Izz3 + 0.4e1 * Iyy3 - 0.4e1 * Izz2 + 0.4e1 * Iyy2 - 0.4e1 * mL * s ^ 2) * phi1p * sin(phi2) * cos(phi2) / 0.4e1 (0.2e1 * m3 * s - m3 * l3 + 0.2e1 * m3 * l2 + 0.2e1 * mL * l2 + 0.2e1 * mL * s) * sp / 0.2e1 phi2p * (0.2e1 * m3 * s - m3 * l3 + 0.2e1 * m3 * l2 + 0.2e1 * mL * l2 + 0.2e1 * mL * s) / 0.2e1; -cos(phi2) ^ 2 * phi1p * (0.2e1 * m3 * s - m3 * l3 + 0.2e1 * m3 * l2 + 0.2e1 * mL * l2 + 0.2e1 * mL * s) / 0.2e1 -phi2p * (0.2e1 * m3 * s - m3 * l3 + 0.2e1 * m3 * l2 + 0.2e1 * mL * l2 + 0.2e1 * mL * s) / 0.2e1 0;];

% vector of gravitational forces
gg = [0 g * (2 * m3 * s - m3 * l3 + 2 * m3 * l2 + l2 * m2 + 2 * mL * l2 + 2 * mL * s) * cos(phi2) / 0.2e1 g * (m3 + mL) * sin(phi2)]';

% dissipative forces
rr = [d1 * phi1p d2 * phi2p d3 * sp]';

% motion equations
qqp=[phi1p,phi2p,sp]';
ttau = [M1 M2 F]';
qqpp=DDinv*(-CC*qqp - gg - rr + ttau);

% define output
xp(1) = phi1p;
xp(2) = phi2p;
xp(3) = sp;
xp(4) = qqpp(1);
xp(5) = qqpp(2);
xp(6) = qqpp(3);

== matlab function Roboter_RRP_Sim/Robotermodell/MATLAB Function1 ==
  data: q output; x input; parSys parameter; qp output; DDdet output
function [q,qp,DDdet] = h(x, parSys)

% define size of the outputs
q     = zeros(3,1);
qp    = zeros(3,1);
DDdet = 0;

% map parameters
m1  = parSys.m1;
m2  = parSys.m2;
m3  = parSys.m3;
mL  = parSys.mL;
l1  = parSys.l1;  
l2  = parSys.l2;  
l3  = parSys.l3;  
Ixx1 = parSys.Ixx1;  
Iyy1 = parSys.Iyy1;    
Izz1 = parSys.Izz1;  
Ixx2 = parSys.Ixx2;    
Iyy2 = parSys.Iyy2;    
Izz2 = parSys.Izz2;    
Ixx3 = parSys.Ixx3;    
Iyy3 = parSys.Iyy3;    
Izz3 = parSys.Izz3;    
d1   = parSys.d1;    
d2   = parSys.d2;    
d3   = parSys.d3; 
g    = parSys.g;

%  map states
phi1  = x(1);
phi2  = x(2);
s     = x(3);
phi1p = x(4);
phi2p = x(5);
sp    = x(6);


% determinant of the mass matrix
DDdet = (((l2 + s - l3 / 0.2e1) ^ 2 * m3 + (m2 / 0.4e1 + mL) * l2 ^ 2 + 0.2e1 * mL * l2 * s - Iyy3 + mL * s ^ 2 + Izz2 - Iyy2 + Izz3) * cos(phi2) ^ 2 + Iyy2 + Iyy3 + Izz1) * ((l2 + s - l3 / 0.2e1) ^ 2 * m3 + (m2 / 0.4e1 + mL) * l2 ^ 2 + 0.2e1 * mL * l2 * s + mL * s ^ 2 + Ixx2 + Ixx3) * (m3 + mL);

% define outputs
q(1) = phi1;
q(2) = phi2;
q(3) = s;

qp(1) = phi1p;
qp(2) = phi2p;
qp(3) = sp;
